simulink model "Maglev_Software"  (R2024a)
settings: Solver=VariableStepAuto  StartTime=0.0  StopTime=1  RelTol=1e-3
values from neighbouring files (symbols this model uses):
  d = data(:,1)    [MagLev_Data(1).m]
undefined symbols (not defined in the file or in its folder): A, B, C, D, n, x0
settings Model: Creator=legom  LastModifiedBy=legom

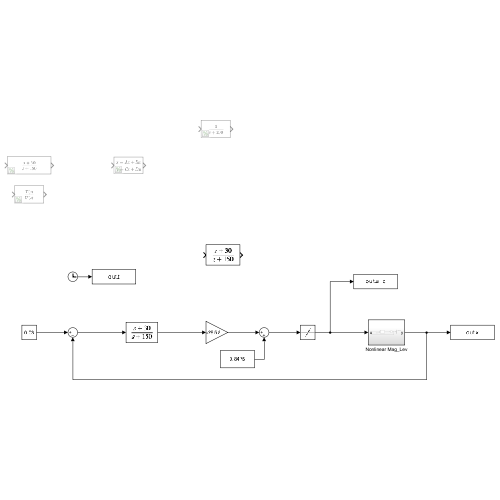
[thumbnail: Simulink's stored preview of the top-level diagram]
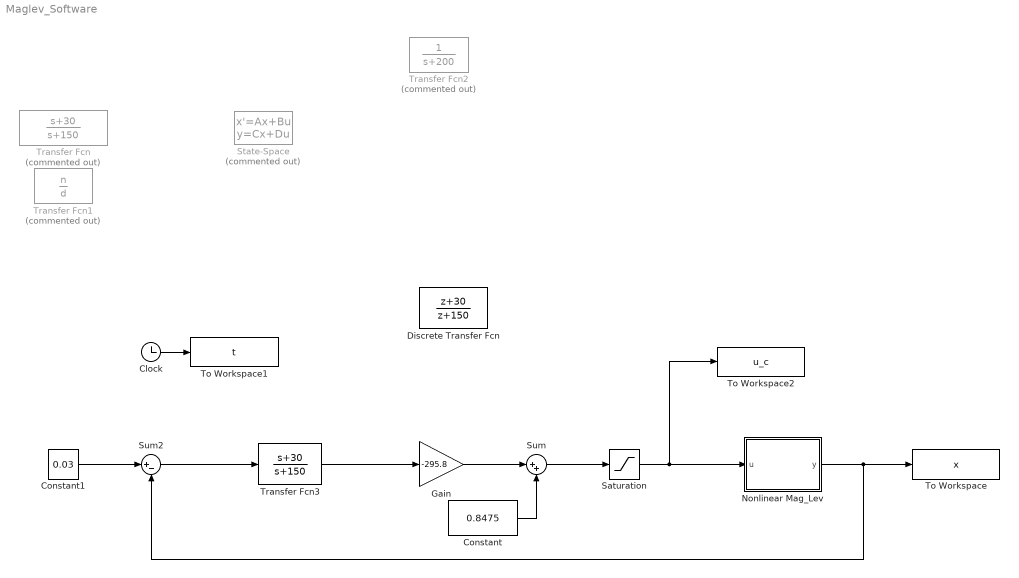
== system Maglev_Software ==
  Clock : Clock
  Constant : Constant  Value=0.8475
  Constant1 : Constant  Value=0.03
  Discrete Transfer Fcn : DiscreteTransferFcn  Numerator=[1 30]  Denominator=[1 150]
  Gain : Gain  Gain=-295.8
  Nonlinear Mag_Lev : Subsystem
  Saturation : Saturate  UpperLimit=3.25  LowerLimit=-3.25
  State-Space : StateSpace  Commented=on  A=A  B=B  C=C  D=D  InitialCondition=[0.025;0;0.25]
  Sum : Sum  Inputs=|++
  Sum2 : Sum  Inputs=|+-
  To Workspace : ToWorkspace  VariableName=x  SampleTime=-1
      settings: Save2DSignal=2-D array (concatenate along first dimension)
  To Workspace1 : ToWorkspace  VariableName=t  SampleTime=-1
      settings: Save2DSignal=2-D array (concatenate along first dimension)
  To Workspace2 : ToWorkspace  VariableName=u_c  SampleTime=-1
      settings: Save2DSignal=2-D array (concatenate along first dimension)
  Transfer Fcn : TransferFcn  Commented=on  Numerator=[1 30]  Denominator=[1 150]
  Transfer Fcn1 : TransferFcn  Commented=on  Numerator=n  Denominator=d
  Transfer Fcn2 : TransferFcn  Commented=on  Denominator=[1 200]
  Transfer Fcn3 : TransferFcn  Numerator=[1 30]  Denominator=[1 150]
  wires:
  Saturation/1 -> Nonlinear Mag_Lev/1(u), To Workspace2/1
  Constant/1 -> Sum/2
  Gain/1 -> Sum/1
  Sum/1 -> Saturation/1
  Clock/1 -> To Workspace1/1
  Constant1/1 -> Sum2/1
  Nonlinear Mag_Lev/1(y) -> Sum2/2, To Workspace/1
  Transfer Fcn3/1 -> Gain/1
  Sum2/1 -> Transfer Fcn3/1

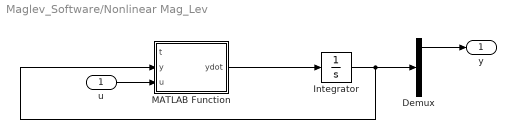
== system Maglev_Software/Nonlinear Mag_Lev ==
  u : Inport
  Demux : Demux  Outputs=3
  Integrator : Integrator  InitialCondition=x0
  MATLAB Function : MATLAB Function  TreatAsAtomicUnit=on
  y : Outport
  wires:
  Integrator/1 -> MATLAB Function/2(y), Demux/1
  u/1 -> MATLAB Function/3(u)
  MATLAB Function/1(ydot) -> Integrator/1
  Demux/1 -> y/1

== matlab function Maglev_Software/Nonlinear Mag_Lev/MATLAB Function ==
  data: t input; y input; u input; ydot output
function ydot  = Mag_Lev(t, y, u)
[ydot] = Mag_Lev(t, y, u);
